simulink model "SIMU_1"  (R2023b)
settings: Solver=VariableStepAuto  StartTime=0.0  StopTime=100  RelTol=1e-3
values from neighbouring files (symbols this model uses):
  p1 = q0*Beta1    [PUNTO_1.m]
  p2 = q0*Beta2    [PUNTO_1.m]
  q0 = 1/(Beta1 + Beta2)    [PUNTO_1.m]
  q1 = q0*alpha1    [PUNTO_1.m]
  q2 = q0*alpha2    [PUNTO_1.m]
  T = 40/20    (= 2)    [PUNTO_1.m]    (also in c2d.m = SE2 * M2)
  T2 = 10/2    (= 5)    [PUNTO_1.m]

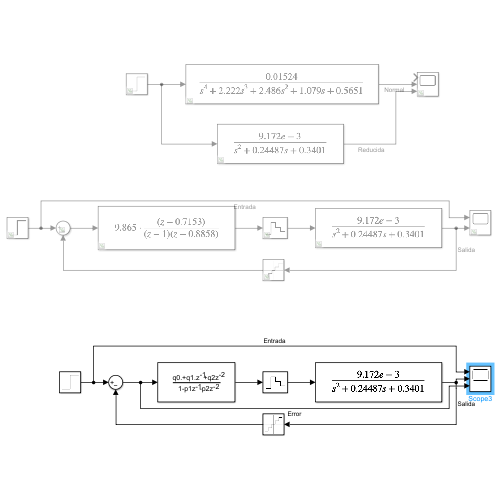
[thumbnail: Simulink's stored preview of the top-level diagram]
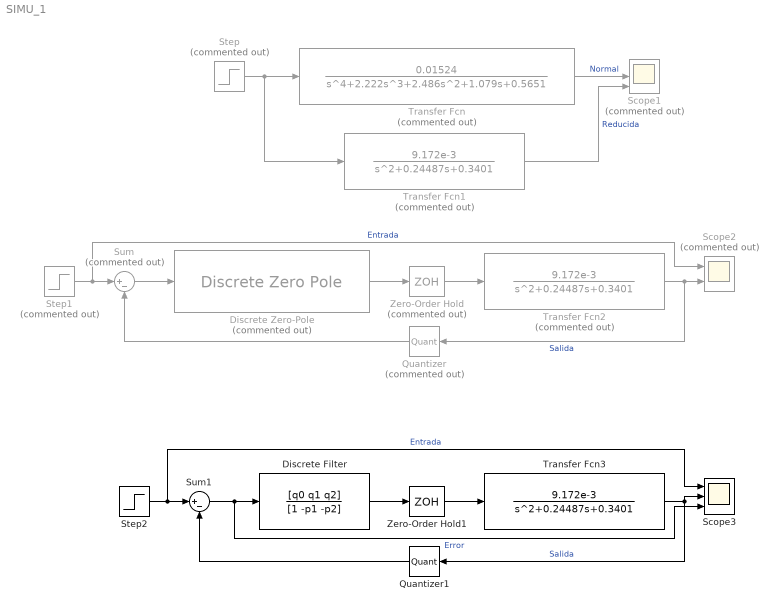
== system SIMU_1 ==
  Discrete Zero-Pole : DiscreteZeroPole  Commented=on  Zeros=[0.7153]  Poles=[1 0.8858]  Gain=9.865  SampleTime=-1
  Discrete Filter : DiscreteFilter  Numerator=[q0 q1 q2]  Denominator=[1 -p1 -p2]
  Quantizer : Quantizer  Commented=on  QuantizationInterval=3.3/(1024-1)
  Quantizer1 : Quantizer  QuantizationInterval=3.3/(1024-1)
  Scope1 : Scope  Commented=on  NumInputPorts=3
  Scope2 : Scope  Commented=on  NumInputPorts=2
  Scope3 : Scope  NumInputPorts=3
  Step : Step  Commented=on  Time=0  SampleTime=0
  Step1 : Step  Commented=on  Time=0  SampleTime=0
  Step2 : Step  Time=0  SampleTime=0
  Sum : Sum  Commented=on  Inputs=|+-
  Sum1 : Sum  Inputs=|+-
  Transfer Fcn : TransferFcn  Commented=on  Numerator=0.01524  Denominator=[1 2.222 2.486 1.079 0.5651]
  Transfer Fcn1 : TransferFcn  Commented=on  Numerator=9.172e-3  Denominator=[1 0.24487 0.3401]
  Transfer Fcn2 : TransferFcn  Commented=on  Numerator=9.172e-3  Denominator=[1 0.24487 0.3401]
  Transfer Fcn3 : TransferFcn  Numerator=9.172e-3  Denominator=[1 0.24487 0.3401]
  Zero-Order Hold : ZeroOrderHold  Commented=on  SampleTime=T
  Zero-Order Hold1 : ZeroOrderHold  SampleTime=T2
  wires:
  Step/1 -> Transfer Fcn1/1, Transfer Fcn/1
  Transfer Fcn/1 -> Scope1/2  "Normal"
  Transfer Fcn1/1 -> Scope1/3  "Reducida"
  Zero-Order Hold/1 -> Transfer Fcn2/1
  Discrete Zero-Pole/1 -> Zero-Order Hold/1
  Transfer Fcn2/1 -> Quantizer/1, Scope2/2  "Salida"
  Step1/1 -> Scope2/1, Sum/1  "Entrada"
  Sum/1 -> Discrete Zero-Pole/1
  Quantizer/1 -> Sum/2
  Quantizer1/1 -> Sum1/2
  Step2/1 -> Scope3/1, Sum1/1  "Entrada"
  Transfer Fcn3/1 -> Quantizer1/1, Scope3/2  "Salida"
  Zero-Order Hold1/1 -> Transfer Fcn3/1
  Sum1/1 -> Scope3/3, Discrete Filter/1  "Error"
  Discrete Filter/1 -> Zero-Order Hold1/1
